simulink model "eq_1_cond_sim"  (R2021a)
settings: Solver=VariableStepAuto  StartTime=0.0  StopTime=10.0  RelTol=1e-3
settings Model: Creator=55189  LastModifiedBy=55189

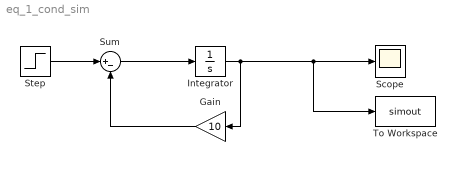
== system eq_1_cond_sim ==
  Gain : Gain  Gain=10
  Integrator : Integrator  InitialCondition=10
  Scope : Scope
  Step : Step  Time=0  After=10  SampleTime=0
  Sum : Sum  Inputs=|+-
  To Workspace : ToWorkspace  VariableName=simout  SampleTime=-1
  wires:
  Sum/1 -> Integrator/1
  Integrator/1 -> Gain/1, To Workspace/1, Scope/1
  Gain/1 -> Sum/2
  Step/1 -> Sum/1
